simulink model "carSimACCLK"  (Simulink 10.2)
settings: Solver=ode23  StartTime=0.0  StopTime=80  FixedStep=1e-3  MaxStep=1e-2  RelTol=1e-3  EnableMultiTasking=on
libraries: simulink x5, dsparch4 x1
settings Model: LogicAnalyzerSignalOrdering=2c38dcc2-2ce4-44d7-bc47-ecfd3f78c9bc,43d34be1-2abe-4690-b550-79d99dd1860e,4a55a25e-455b-4f1c-be2e-1f375bbe41e4,4b197a40-1570-45d4-a952-fe9de0dc1ab5,12be2a9c-a868-4901-9855-7311f94e1c65,7a3363cb-5b35-4870-a861-6749fa4c6c84,d5c23654-3a48-4008-a3e4-0f09cca63f01,db4552fa-7eaf-453d-b285-63f4f7b0a5f4,005b0ed1-16df-4a19-95da-62a42ccf9ea3  Creator=hp  LastModifiedBy=11634
settings SolverCC: AlgebraicLoopSolver=LineSearch
settings DataIOCC: LimitDataPoints=on  SignalLoggingName=sigsOut
settings OptimizationCC: ExpressionDepthLimit=2147483647  InitFltsAndDblsToZero=on
settings DebuggingCC: SaveWithParameterizedLinksMsg=none  SignalResolutionControl=TryResolveAllWithWarning  MultiTaskDSMMsg=warning  MultiTaskCondExecSysMsg=none  StateNameClashWarn=warning
settings HardwareCC: TargetUnknown=on
settings GRTTargetCC: TargetFcnLib=ansi_tfl_tmw.mat

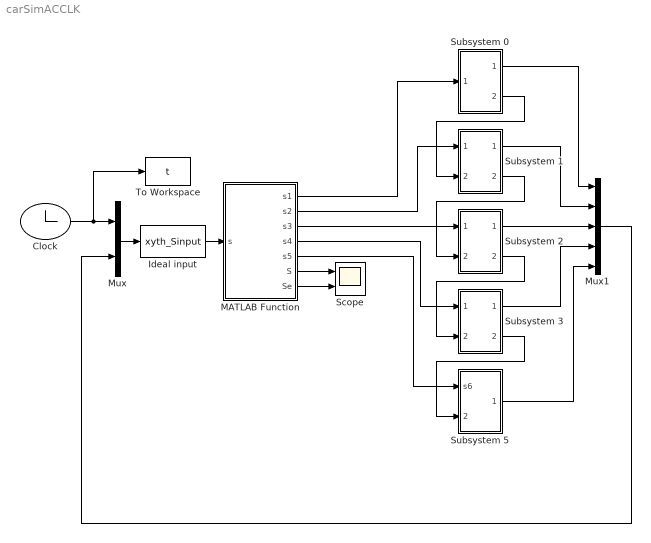
== system carSimACCLK ==
  Clock : Clock
  Ideal input : S-Function  FunctionName=xyth_Sinput  SFunctionDeploymentMode=off  EnableBusSupport=off
  MATLAB Function : MATLAB Function  TreatAsAtomicUnit=on
  Mux : Mux  Inputs=2
  Mux1 : Mux  Inputs=5
  Scope : Scope  NumInputPorts=2
  Subsystem 0 : Subsystem
  Subsystem 1 : Subsystem
  Subsystem 2 : Subsystem
  Subsystem 3 : Subsystem
  Subsystem 5 : Subsystem
  To Workspace : ToWorkspace  VariableName=t  SampleTime=-1
  wires:
  Clock/1 -> To Workspace/1, Mux/1
  Mux/1 -> Ideal input/1
  Ideal input/1 -> MATLAB Function/1(s)
  MATLAB Function/6(S) -> Scope/1
  MATLAB Function/7(Se) -> Scope/2
  MATLAB Function/2(s2) -> Subsystem 1/1(In1)
  Subsystem 1/1(Out1) -> Mux1/2
  MATLAB Function/1(s1) -> Subsystem 0/1(In1)
  Subsystem 0/1(Out1) -> Mux1/1
  Subsystem 0/2(Out2) -> Subsystem 1/2(In2)
  Subsystem 5/1(Out1) -> Mux1/5
  Mux1/1 -> Mux/2
  Subsystem 2/2(Out2) -> Subsystem 3/2(In2)
  Subsystem 2/1(Out1) -> Mux1/3
  Subsystem 3/1(Out1) -> Mux1/4
  MATLAB Function/4(s4) -> Subsystem 3/1(1)
  MATLAB Function/3(s3) -> Subsystem 2/1(In1)
  Subsystem 1/2(2) -> Subsystem 2/2(2)
  Subsystem 3/2(Out2) -> Subsystem 5/2(In2)
  MATLAB Function/5(s5) -> Subsystem 5/1(s6)

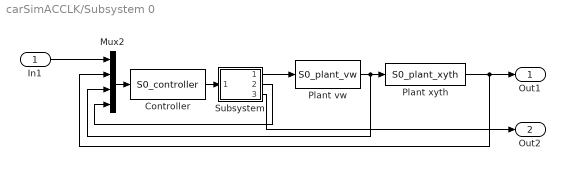
== system carSimACCLK/Subsystem 0 ==
  In1 : Inport
  Controller : S-Function  FunctionName=S0_controller  SFunctionDeploymentMode=off  EnableBusSupport=off
  Mux2 : Mux
  Plant vw : S-Function  FunctionName=S0_plant_vw  SFunctionDeploymentMode=off  EnableBusSupport=off
  Plant xyth : S-Function  FunctionName=S0_plant_xyth  SFunctionDeploymentMode=off  EnableBusSupport=off
  Subsystem : Subsystem
  Out1 : Outport
  Out2 : Outport  Port=2
  wires:
  Subsystem/1(Out1) -> Plant vw/1
  Subsystem/2(Out2) -> Mux2/4
  Subsystem/3(Out3) -> Out2/1
  Plant xyth/1 -> Mux2/2, Out1/1
  Mux2/1 -> Controller/1
  In1/1 -> Mux2/1
  Plant vw/1 -> Mux2/3, Plant xyth/1
  Controller/1 -> Subsystem/1(In1)

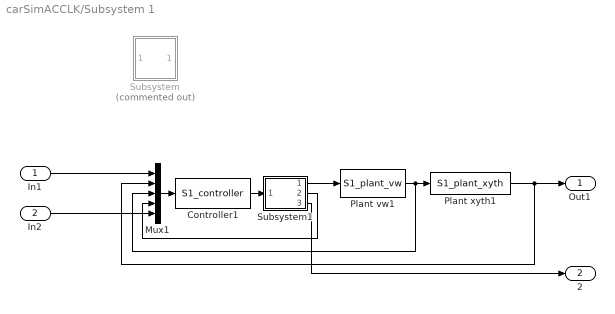
== system carSimACCLK/Subsystem 1 ==
  In1 : Inport
  In2 : Inport  Port=2
  Controller1 : S-Function  FunctionName=S1_controller  SFunctionDeploymentMode=off  EnableBusSupport=off
  Mux1 : Mux  Inputs=5
  Plant vw1 : S-Function  FunctionName=S1_plant_vw  SFunctionDeploymentMode=off  EnableBusSupport=off
  Plant xyth1 : S-Function  FunctionName=S1_plant_xyth  SFunctionDeploymentMode=off  EnableBusSupport=off
  Subsystem : Subsystem  Commented=on
  Subsystem1 : Subsystem
  Out1 : Outport
  2 : Outport  Port=2
  wires:
  Plant xyth1/1 -> Mux1/2, Out1/1
  In2/1 -> Mux1/5
  Plant vw1/1 -> Mux1/3, Plant xyth1/1
  Subsystem1/3(Out3) -> 2/1
  Subsystem1/1(Out1) -> Plant vw1/1
  Mux1/1 -> Controller1/1
  Controller1/1 -> Subsystem1/1(In1)
  Subsystem1/2(Out2) -> Mux1/4
  In1/1 -> Mux1/1

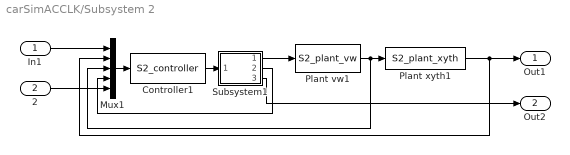
== system carSimACCLK/Subsystem 2 ==
  In1 : Inport
  2 : Inport  Port=2
  Controller1 : S-Function  FunctionName=S2_controller  SFunctionDeploymentMode=off  EnableBusSupport=off
  Mux1 : Mux  Inputs=5
  Plant vw1 : S-Function  FunctionName=S2_plant_vw  SFunctionDeploymentMode=off  EnableBusSupport=off
  Plant xyth1 : S-Function  FunctionName=S2_plant_xyth  SFunctionDeploymentMode=off  EnableBusSupport=off
  Subsystem1 : Subsystem
  Out1 : Outport
  Out2 : Outport  Port=2
  wires:
  Subsystem1/2(Out2) -> Mux1/4
  Controller1/1 -> Subsystem1/1(In1)
  Mux1/1 -> Controller1/1
  Subsystem1/1(Out1) -> Plant vw1/1
  Subsystem1/3(Out3) -> Out2/1
  Plant vw1/1 -> Mux1/3, Plant xyth1/1
  2/1 -> Mux1/5
  In1/1 -> Mux1/1
  Plant xyth1/1 -> Mux1/2, Out1/1

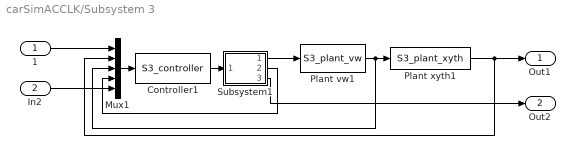
== system carSimACCLK/Subsystem 3 ==
  1 : Inport
  In2 : Inport  Port=2
  Controller1 : S-Function  FunctionName=S3_controller  SFunctionDeploymentMode=off  EnableBusSupport=off
  Mux1 : Mux  Inputs=5
  Plant vw1 : S-Function  FunctionName=S3_plant_vw  SFunctionDeploymentMode=off  EnableBusSupport=off
  Plant xyth1 : S-Function  FunctionName=S3_plant_xyth  SFunctionDeploymentMode=off  EnableBusSupport=off
  Subsystem1 : Subsystem
  Out1 : Outport
  Out2 : Outport  Port=2
  wires:
  Plant xyth1/1 -> Mux1/2, Out1/1
  1/1 -> Mux1/1
  In2/1 -> Mux1/5
  Plant vw1/1 -> Plant xyth1/1, Mux1/3
  Subsystem1/3(Out3) -> Out2/1
  Subsystem1/1(Out1) -> Plant vw1/1
  Mux1/1 -> Controller1/1
  Controller1/1 -> Subsystem1/1(In1)
  Subsystem1/2(Out2) -> Mux1/4

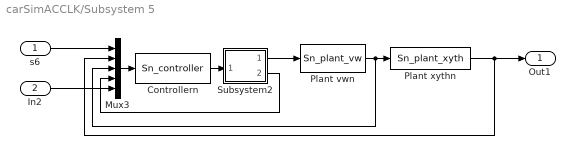
== system carSimACCLK/Subsystem 5 ==
  s6 : Inport
  In2 : Inport  Port=2
  Controllern : S-Function  FunctionName=Sn_controller  SFunctionDeploymentMode=off  EnableBusSupport=off
  Mux3 : Mux  Inputs=5
  Plant vwn : S-Function  FunctionName=Sn_plant_vw  SFunctionDeploymentMode=off  EnableBusSupport=off
  Plant xythn : S-Function  FunctionName=Sn_plant_xyth  SFunctionDeploymentMode=off  EnableBusSupport=off
  Subsystem2 : Subsystem
  Out1 : Outport
  wires:
  Subsystem2/1(Out1) -> Plant vwn/1
  Subsystem2/2(Out2) -> Mux3/4
  Mux3/1 -> Controllern/1
  Plant vwn/1 -> Mux3/3, Plant xythn/1
  Controllern/1 -> Subsystem2/1(In1)
  In2/1 -> Mux3/5
  Plant xythn/1 -> Mux3/2, Out1/1
  s6/1 -> Mux3/1

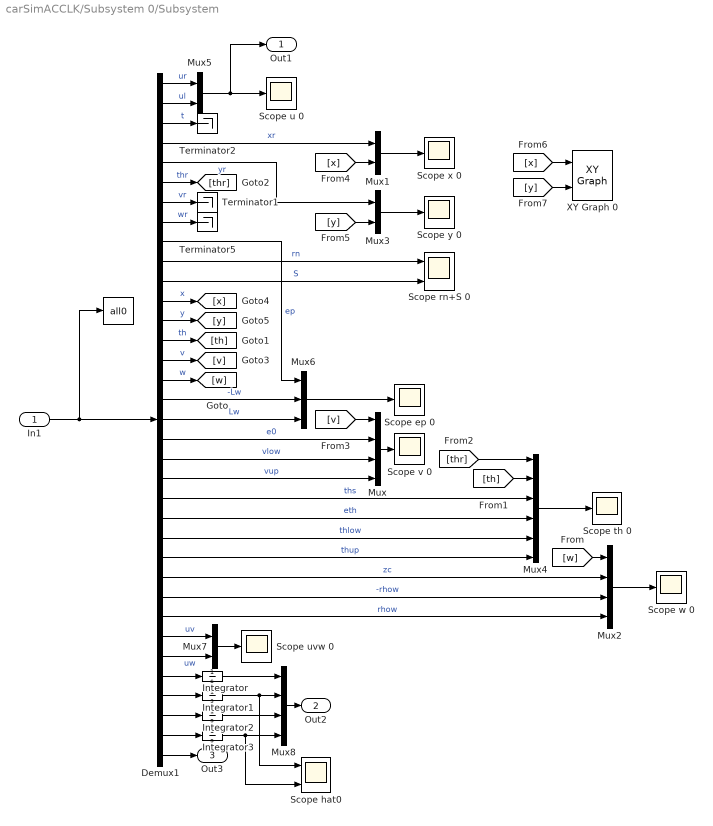
== system carSimACCLK/Subsystem 0/Subsystem ==
  In1 : Inport
  " " : ToWorkspace  VariableName=all0  SampleTime=-1
  Demux1 : Demux  Outputs=35
  Integrator : Integrator
  Integrator1 : Integrator  InitialCondition=0.1
  Integrator2 : Integrator
  Integrator3 : Integrator  InitialCondition=0.1
  Mux : Mux
  Mux{1,3,5,7} (4 alike) : Mux  Inputs=2
  Mux2 : Mux
  Mux4 : Mux  Inputs=6
  Mux6 : Mux  Inputs=3
  Mux8 : Mux
  Scope ep 0 : Scope
  Scope hat0 : Scope  NumInputPorts=2
  Scope rn+S 0 : Scope  NumInputPorts=2
  Scope th 0 : Scope
  Scope u 0 : Scope
  Scope uvw 0 : Scope
  Scope v 0 : Scope
  Scope w 0 : Scope
  Scope x 0 : Scope
  Scope y 0 : Scope
  Terminator1 : Terminator
  Terminator2 : Terminator
  Terminator5 : Terminator
  XY Graph 0 : simulink/Sinks/XY Graph  xmin=-400  xmax=400  ymin=-400  ymax=400  st=-1
  Out1 : Outport
  Out2 : Outport  Port=2
  Out3 : Outport  Port=3
  wires:
  In1/1 -> " "/1, Demux1/1
  Demux1/2 -> Mux5/2  "ul"
  Mux5/1 -> Scope u 0/1, Out1/1
  Demux1/1 -> Mux5/1  "ur"
  Mux3/1 -> Scope y 0/1
  Mux1/1 -> Scope x 0/1
  Demux1/6 -> [thr]  "thr"
  Demux1/8 -> Terminator5/1  "wr"
  Demux1/7 -> Terminator1/1  "vr"
  Demux1/3 -> Terminator2/1  "t"
  Demux1/4 -> Mux1/1  "xr"
  Demux1/5 -> Mux3/1  "yr"
  [x] -> Mux1/2
  [y] -> Mux3/2
  [x] -> XY Graph 0/1
  [y] -> XY Graph 0/2
  Demux1/10 -> Scope rn+S 0/1  "rn"
  Mux/1 -> Scope v 0/1
  Mux2/1 -> Scope w 0/1
  [w] -> Mux2/1
  [th] -> Mux4/2
  Mux6/1 -> Scope ep 0/1
  [thr] -> Mux4/1
  Demux1/13 -> [y]  "y"
  Demux1/28 -> Mux2/4  "rhow"
  Mux7/1 -> Scope uvw 0/1
  Demux1/29 -> Mux7/1  "uv"
  Demux1/12 -> [x]  "x"
  Demux1/15 -> [v]  "v"
  Demux1/14 -> [th]  "th"
  Demux1/17 -> Mux6/2  "-Lw"
  Demux1/27 -> Mux2/3  "-rhow"
  [v] -> Mux/1
  Demux1/26 -> Mux2/2  "zc"
  Demux1/22 -> Mux4/3  "ths"
  Demux1/23 -> Mux4/4  "eth"
  Demux1/19 -> Mux/2  "e0"
  Demux1/21 -> Mux/4  "vup"
  Demux1/16 -> [w]  "w"
  Demux1/25 -> Mux4/6  "thup"
  Demux1/24 -> Mux4/5  "thlow"
  Demux1/30 -> Mux7/2  "uw"
  Mux4/1 -> Scope th 0/1
  Demux1/20 -> Mux/3  "vlow"
  Demux1/9 -> Mux6/1  "ep"
  Demux1/18 -> Mux6/3  "Lw"
  Demux1/11 -> Scope rn+S 0/2  "S"
  Mux8/1 -> Out2/1
  Demux1/31 -> Integrator/1
  Demux1/32 -> Integrator1/1
  Integrator1/1 -> Mux8/2, Scope hat0/1
  Integrator/1 -> Mux8/1
  Integrator2/1 -> Mux8/3
  Demux1/33 -> Integrator2/1
  Integrator3/1 -> Mux8/4, Scope hat0/2
  Demux1/34 -> Integrator3/1
  Demux1/35 -> Out3/1

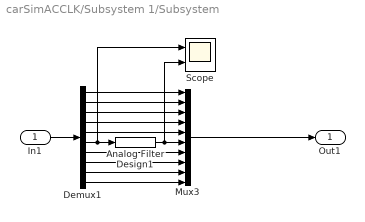
== system carSimACCLK/Subsystem 1/Subsystem ==
  In1 : Inport
  Analog Filter Design1 : dsparch4/Analog Filter Design  method=Butterworth  filttype=Lowpass  N=8  Wlo=50  Whi=80  Rp=2  Rs=40
  Demux1 : Demux  Outputs=10
  Mux3 : Mux  Inputs=10
  Scope : Scope  NumInputPorts=2
  Out1 : Outport
  wires:
  Demux1/1 -> Mux3/1
  Analog Filter Design1/1 -> Scope/2, Mux3/6
  Demux1/7 -> Mux3/7
  Mux3/1 -> Out1/1
  Demux1/4 -> Mux3/4
  Demux1/9 -> Mux3/9
  In1/1 -> Demux1/1
  Demux1/2 -> Mux3/2
  Demux1/3 -> Mux3/3
  Demux1/5 -> Mux3/5
  Demux1/10 -> Mux3/10
  Demux1/8 -> Mux3/8
  Demux1/6 -> Scope/1, Analog Filter Design1/1

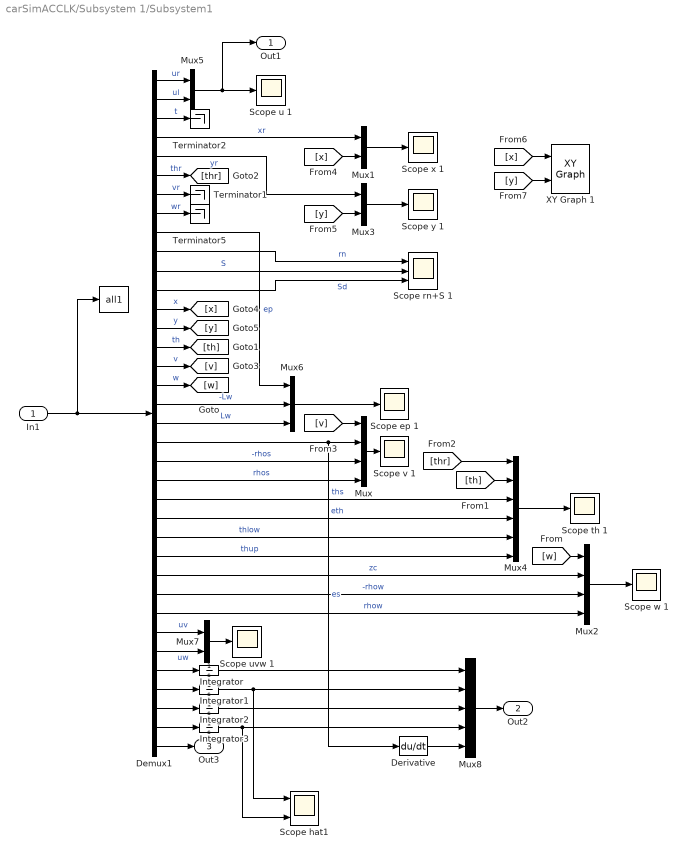
== system carSimACCLK/Subsystem 1/Subsystem1 ==
  In1 : Inport
  " " : ToWorkspace  VariableName=all1  SampleTime=-1
  Demux1 : Demux  Outputs=36
  Derivative : Derivative
  Integrator : Integrator
  Integrator1 : Integrator  InitialCondition=0.1
  Integrator2 : Integrator
  Integrator3 : Integrator  InitialCondition=0.1
  Mux : Mux
  Mux{1,3,5,7} (4 alike) : Mux  Inputs=2
  Mux2 : Mux
  Mux4 : Mux  Inputs=6
  Mux6 : Mux  Inputs=3
  Mux8 : Mux  Inputs=5
  Scope ep 1 : Scope
  Scope hat1 : Scope  NumInputPorts=2
  Scope rn+S 1 : Scope  NumInputPorts=3
  Scope th 1 : Scope
  Scope u 1 : Scope
  Scope uvw 1 : Scope
  Scope v 1 : Scope
  Scope w 1 : Scope
  Scope x 1 : Scope
  Scope y 1 : Scope
  Terminator1 : Terminator
  Terminator2 : Terminator
  Terminator5 : Terminator
  XY Graph 1 : simulink/Sinks/XY Graph  xmin=-400  xmax=400  ymin=-400  ymax=400  st=-1
  Out1 : Outport
  Out2 : Outport  Port=2
  Out3 : Outport  Port=3
  wires:
  Demux1/11 -> Scope rn+S 1/2  "S"
  Demux1/13 -> [x]  "x"
  Demux1/10 -> Scope rn+S 1/1  "rn"
  [y] -> XY Graph 1/2
  [x] -> XY Graph 1/1
  [y] -> Mux3/2
  [x] -> Mux1/2
  Demux1/5 -> Mux3/1  "yr"
  Demux1/4 -> Mux1/1  "xr"
  Demux1/3 -> Terminator2/1  "t"
  Demux1/7 -> Terminator1/1  "vr"
  Demux1/8 -> Terminator5/1  "wr"
  Demux1/6 -> [thr]  "thr"
  Mux1/1 -> Scope x 1/1
  Mux3/1 -> Scope y 1/1
  Demux1/1 -> Mux5/1  "ur"
  Mux5/1 -> Out1/1, Scope u 1/1
  Demux1/2 -> Mux5/2  "ul"
  In1/1 -> " "/1, Demux1/1
  Demux1/18 -> Mux6/2  "-Lw"
  Mux4/1 -> Scope th 1/1
  Mux/1 -> Scope v 1/1
  Demux1/30 -> Mux7/1  "uv"
  [w] -> Mux2/1
  [th] -> Mux4/2
  Demux1/16 -> [v]  "v"
  Mux6/1 -> Scope ep 1/1
  [thr] -> Mux4/1
  Demux1/21 -> Mux/3  "-rhos"
  Demux1/15 -> [th]  "th"
  [v] -> Mux/1
  Demux1/23 -> Mux4/3  "ths"
  Demux1/20 -> Mux/2, Derivative/1  "es"
  Demux1/25 -> Mux4/5  "thlow"
  Demux1/22 -> Mux/4  "rhos"
  Demux1/28 -> Mux2/3  "-rhow"
  Demux1/31 -> Mux7/2  "uw"
  Demux1/27 -> Mux2/2  "zc"
  Demux1/17 -> [w]  "w"
  Demux1/26 -> Mux4/6  "thup"
  Demux1/29 -> Mux2/4  "rhow"
  Demux1/19 -> Mux6/3  "Lw"
  Demux1/24 -> Mux4/4  "eth"
  Demux1/9 -> Mux6/1  "ep"
  Mux2/1 -> Scope w 1/1
  Mux7/1 -> Scope uvw 1/1
  Demux1/14 -> [y]  "y"
  Demux1/12 -> Scope rn+S 1/3  "Sd"
  Mux8/1 -> Out2/1
  Integrator/1 -> Mux8/1
  Demux1/32 -> Integrator/1
  Demux1/33 -> Integrator1/1
  Integrator1/1 -> Scope hat1/1, Mux8/2
  Demux1/36 -> Out3/1
  Demux1/34 -> Integrator2/1
  Demux1/35 -> Integrator3/1
  Integrator2/1 -> Mux8/3
  Integrator3/1 -> Scope hat1/2, Mux8/4
  Derivative/1 -> Mux8/5

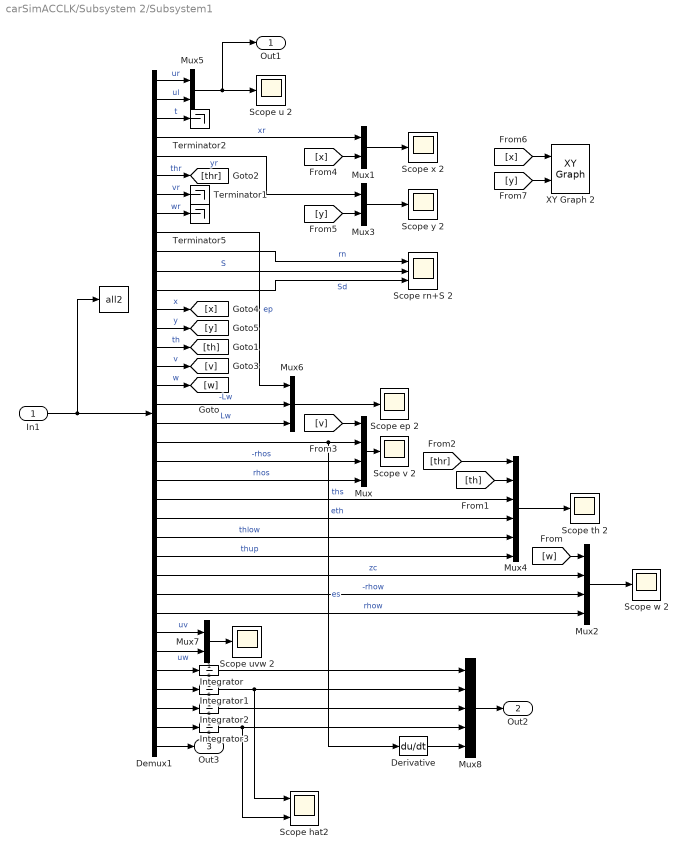
== system carSimACCLK/Subsystem 2/Subsystem1 ==
  In1 : Inport
  " " : ToWorkspace  VariableName=all2  SampleTime=-1
  Demux1 : Demux  Outputs=36
  Derivative : Derivative
  Integrator : Integrator
  Integrator1 : Integrator  InitialCondition=0.1
  Integrator2 : Integrator
  Integrator3 : Integrator  InitialCondition=0.1
  Mux : Mux
  Mux{1,3,5,7} (4 alike) : Mux  Inputs=2
  Mux2 : Mux
  Mux4 : Mux  Inputs=6
  Mux6 : Mux  Inputs=3
  Mux8 : Mux  Inputs=5
  Scope ep 2 : Scope
  Scope hat2 : Scope  NumInputPorts=2
  Scope rn+S 2 : Scope  NumInputPorts=3
  Scope th 2 : Scope
  Scope u 2 : Scope
  Scope uvw 2 : Scope
  Scope v 2 : Scope
  Scope w 2 : Scope
  Scope x 2 : Scope
  Scope y 2 : Scope
  Terminator1 : Terminator
  Terminator2 : Terminator
  Terminator5 : Terminator
  XY Graph 2 : simulink/Sinks/XY Graph  xmin=-400  xmax=400  ymin=-400  ymax=400  st=-1
  Out1 : Outport
  Out2 : Outport  Port=2
  Out3 : Outport  Port=3
  wires:
  Derivative/1 -> Mux8/5
  Integrator3/1 -> Mux8/4, Scope hat2/2
  Integrator2/1 -> Mux8/3
  Demux1/35 -> Integrator3/1
  Demux1/34 -> Integrator2/1
  Demux1/36 -> Out3/1
  Integrator1/1 -> Scope hat2/1, Mux8/2
  Demux1/33 -> Integrator1/1
  Demux1/32 -> Integrator/1
  Integrator/1 -> Mux8/1
  Mux8/1 -> Out2/1
  Demux1/12 -> Scope rn+S 2/3  "Sd"
  Demux1/14 -> [y]  "y"
  Mux7/1 -> Scope uvw 2/1
  Mux2/1 -> Scope w 2/1
  Demux1/9 -> Mux6/1  "ep"
  Demux1/24 -> Mux4/4  "eth"
  Demux1/19 -> Mux6/3  "Lw"
  Demux1/29 -> Mux2/4  "rhow"
  Demux1/26 -> Mux4/6  "thup"
  Demux1/17 -> [w]  "w"
  Demux1/27 -> Mux2/2  "zc"
  Demux1/31 -> Mux7/2  "uw"
  Demux1/28 -> Mux2/3  "-rhow"
  Demux1/22 -> Mux/4  "rhos"
  Demux1/25 -> Mux4/5  "thlow"
  Demux1/20 -> Derivative/1, Mux/2  "es"
  Demux1/23 -> Mux4/3  "ths"
  [v] -> Mux/1
  Demux1/15 -> [th]  "th"
  Demux1/21 -> Mux/3  "-rhos"
  [thr] -> Mux4/1
  Mux6/1 -> Scope ep 2/1
  Demux1/16 -> [v]  "v"
  [th] -> Mux4/2
  [w] -> Mux2/1
  Demux1/30 -> Mux7/1  "uv"
  Mux/1 -> Scope v 2/1
  Mux4/1 -> Scope th 2/1
  Demux1/18 -> Mux6/2  "-Lw"
  In1/1 -> Demux1/1, " "/1
  Demux1/2 -> Mux5/2  "ul"
  Mux5/1 -> Scope u 2/1, Out1/1
  Demux1/1 -> Mux5/1  "ur"
  Mux3/1 -> Scope y 2/1
  Mux1/1 -> Scope x 2/1
  Demux1/6 -> [thr]  "thr"
  Demux1/8 -> Terminator5/1  "wr"
  Demux1/7 -> Terminator1/1  "vr"
  Demux1/3 -> Terminator2/1  "t"
  Demux1/4 -> Mux1/1  "xr"
  Demux1/5 -> Mux3/1  "yr"
  [x] -> Mux1/2
  [y] -> Mux3/2
  [x] -> XY Graph 2/1
  [y] -> XY Graph 2/2
  Demux1/10 -> Scope rn+S 2/1  "rn"
  Demux1/13 -> [x]  "x"
  Demux1/11 -> Scope rn+S 2/2  "S"

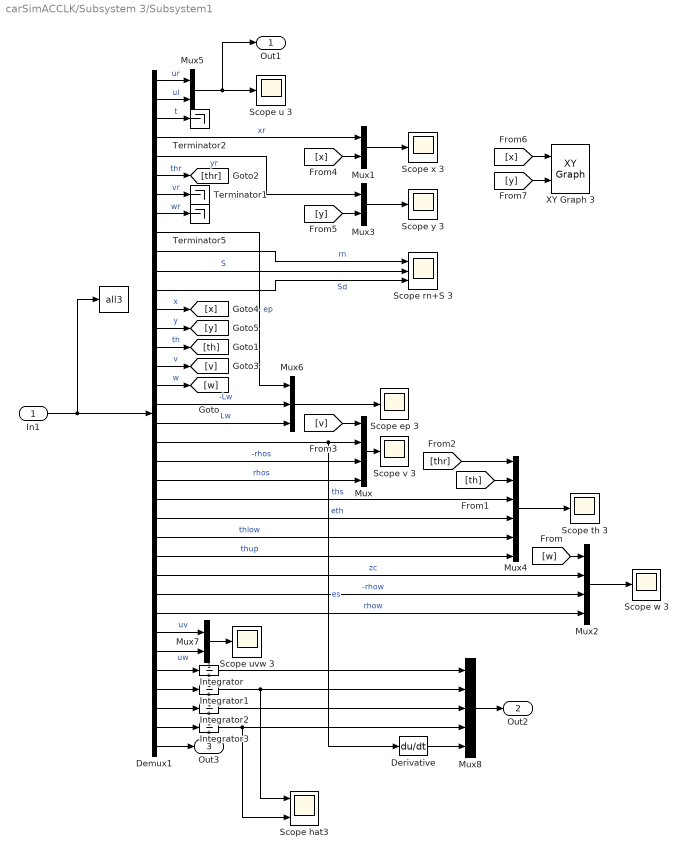
== system carSimACCLK/Subsystem 3/Subsystem1 ==
  In1 : Inport
  " " : ToWorkspace  VariableName=all3  SampleTime=-1
  Demux1 : Demux  Outputs=36
  Derivative : Derivative
  Integrator : Integrator
  Integrator1 : Integrator  InitialCondition=0.1
  Integrator2 : Integrator
  Integrator3 : Integrator  InitialCondition=0.1
  Mux : Mux
  Mux{1,3,5,7} (4 alike) : Mux  Inputs=2
  Mux2 : Mux
  Mux4 : Mux  Inputs=6
  Mux6 : Mux  Inputs=3
  Mux8 : Mux  Inputs=5
  Scope ep 3 : Scope
  Scope hat3 : Scope  NumInputPorts=2
  Scope rn+S 3 : Scope  NumInputPorts=3
  Scope th 3 : Scope
  Scope u 3 : Scope
  Scope uvw 3 : Scope
  Scope v 3 : Scope
  Scope w 3 : Scope
  Scope x 3 : Scope
  Scope y 3 : Scope
  Terminator1 : Terminator
  Terminator2 : Terminator
  Terminator5 : Terminator
  XY Graph 3 : simulink/Sinks/XY Graph  xmin=-400  xmax=400  ymin=-400  ymax=400  st=-1
  Out1 : Outport
  Out2 : Outport  Port=2
  Out3 : Outport  Port=3
  wires:
  Demux1/11 -> Scope rn+S 3/2  "S"
  Demux1/13 -> [x]  "x"
  Demux1/10 -> Scope rn+S 3/1  "rn"
  [y] -> XY Graph 3/2
  [x] -> XY Graph 3/1
  [y] -> Mux3/2
  [x] -> Mux1/2
  Demux1/5 -> Mux3/1  "yr"
  Demux1/4 -> Mux1/1  "xr"
  Demux1/3 -> Terminator2/1  "t"
  Demux1/7 -> Terminator1/1  "vr"
  Demux1/8 -> Terminator5/1  "wr"
  Demux1/6 -> [thr]  "thr"
  Mux1/1 -> Scope x 3/1
  Mux3/1 -> Scope y 3/1
  Demux1/1 -> Mux5/1  "ur"
  Mux5/1 -> Out1/1, Scope u 3/1
  Demux1/2 -> Mux5/2  "ul"
  In1/1 -> " "/1, Demux1/1
  Demux1/18 -> Mux6/2  "-Lw"
  Mux4/1 -> Scope th 3/1
  Mux/1 -> Scope v 3/1
  Demux1/30 -> Mux7/1  "uv"
  [w] -> Mux2/1
  [th] -> Mux4/2
  Demux1/16 -> [v]  "v"
  Mux6/1 -> Scope ep 3/1
  [thr] -> Mux4/1
  Demux1/21 -> Mux/3  "-rhos"
  Demux1/15 -> [th]  "th"
  [v] -> Mux/1
  Demux1/23 -> Mux4/3  "ths"
  Demux1/20 -> Mux/2, Derivative/1  "es"
  Demux1/25 -> Mux4/5  "thlow"
  Demux1/22 -> Mux/4  "rhos"
  Demux1/28 -> Mux2/3  "-rhow"
  Demux1/31 -> Mux7/2  "uw"
  Demux1/27 -> Mux2/2  "zc"
  Demux1/17 -> [w]  "w"
  Demux1/26 -> Mux4/6  "thup"
  Demux1/29 -> Mux2/4  "rhow"
  Demux1/19 -> Mux6/3  "Lw"
  Demux1/24 -> Mux4/4  "eth"
  Demux1/9 -> Mux6/1  "ep"
  Mux2/1 -> Scope w 3/1
  Mux7/1 -> Scope uvw 3/1
  Demux1/14 -> [y]  "y"
  Demux1/12 -> Scope rn+S 3/3  "Sd"
  Mux8/1 -> Out2/1
  Integrator/1 -> Mux8/1
  Demux1/32 -> Integrator/1
  Demux1/33 -> Integrator1/1
  Integrator1/1 -> Scope hat3/1, Mux8/2
  Demux1/36 -> Out3/1
  Demux1/34 -> Integrator2/1
  Demux1/35 -> Integrator3/1
  Integrator2/1 -> Mux8/3
  Integrator3/1 -> Scope hat3/2, Mux8/4
  Derivative/1 -> Mux8/5

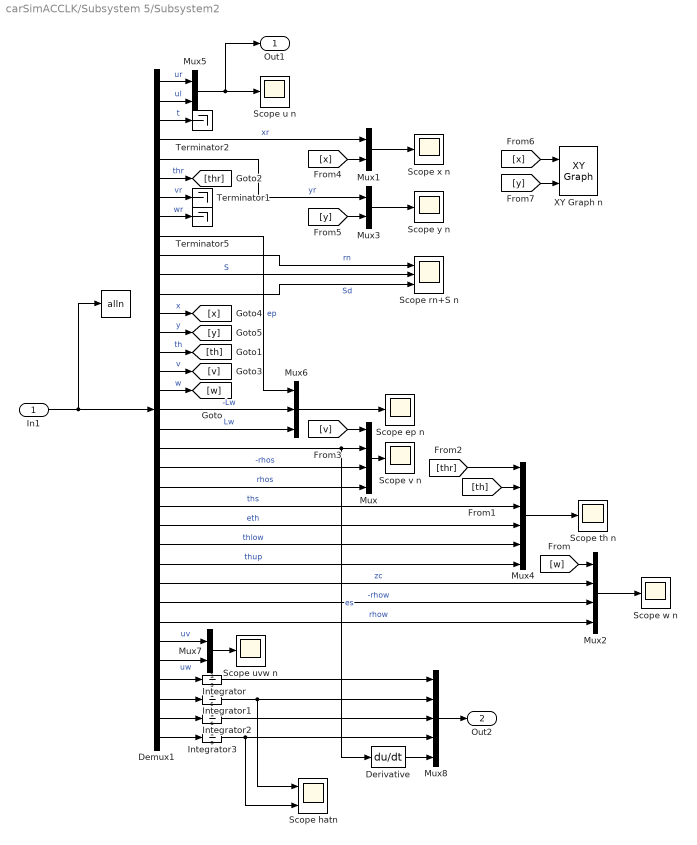
== system carSimACCLK/Subsystem 5/Subsystem2 ==
  In1 : Inport
  " " : ToWorkspace  VariableName=alln  SampleTime=-1
  Demux1 : Demux  Outputs=35
  Derivative : Derivative
  Integrator : Integrator
  Integrator1 : Integrator  InitialCondition=0.1
  Integrator2 : Integrator
  Integrator3 : Integrator  InitialCondition=0.1
  Mux : Mux
  Mux{1,3,5,7} (4 alike) : Mux  Inputs=2
  Mux2 : Mux
  Mux4 : Mux  Inputs=6
  Mux6 : Mux  Inputs=3
  Mux8 : Mux  Inputs=5
  Scope ep n : Scope
  Scope hatn : Scope  NumInputPorts=2
  Scope rn+S n : Scope  NumInputPorts=3
  Scope th n : Scope
  Scope u n : Scope
  Scope uvw n : Scope
  Scope v n : Scope
  Scope w n : Scope
  Scope x n : Scope
  Scope y n : Scope
  Terminator1 : Terminator
  Terminator2 : Terminator
  Terminator5 : Terminator
  XY Graph n : simulink/Sinks/XY Graph  xmin=-400  xmax=400  ymin=-400  ymax=400  st=-1
  Out1 : Outport
  Out2 : Outport  Port=2
  wires:
  In1/1 -> " "/1, Demux1/1
  Demux1/2 -> Mux5/2  "ul"
  Mux5/1 -> Scope u n/1, Out1/1
  Demux1/1 -> Mux5/1  "ur"
  Mux3/1 -> Scope y n/1
  Mux1/1 -> Scope x n/1
  Demux1/6 -> [thr]  "thr"
  Demux1/8 -> Terminator5/1  "wr"
  Demux1/7 -> Terminator1/1  "vr"
  Demux1/3 -> Terminator2/1  "t"
  Demux1/4 -> Mux1/1  "xr"
  Demux1/5 -> Mux3/1  "yr"
  [x] -> Mux1/2
  [y] -> Mux3/2
  [x] -> XY Graph n/1
  [y] -> XY Graph n/2
  Demux1/10 -> Scope rn+S n/1  "rn"
  Demux1/11 -> Scope rn+S n/2  "S"
  Mux7/1 -> Scope uvw n/1
  Demux1/14 -> [y]  "y"
  Demux1/25 -> Mux4/5  "thlow"
  Mux/1 -> Scope v n/1
  Demux1/9 -> Mux6/1  "ep"
  [th] -> Mux4/2
  Demux1/21 -> Mux/3  "-rhos"
  Mux4/1 -> Scope th n/1
  Demux1/26 -> Mux4/6  "thup"
  Demux1/22 -> Mux/4  "rhos"
  Demux1/27 -> Mux2/2  "zc"
  Demux1/17 -> [w]  "w"
  Demux1/24 -> Mux4/4  "eth"
  [v] -> Mux/1
  [thr] -> Mux4/1
  Demux1/23 -> Mux4/3  "ths"
  Demux1/30 -> Mux7/1  "uv"
  Demux1/19 -> Mux6/3  "Lw"
  Mux2/1 -> Scope w n/1
  Demux1/31 -> Mux7/2  "uw"
  Demux1/16 -> [v]  "v"
  [w] -> Mux2/1
  Demux1/15 -> [th]  "th"
  Demux1/13 -> [x]  "x"
  Demux1/20 -> Derivative/1, Mux/2  "es"
  Demux1/29 -> Mux2/4  "rhow"
  Integrator1/1 -> Scope hatn/1, Mux8/2
  Integrator/1 -> Mux8/1
  Demux1/18 -> Mux6/2  "-Lw"
  Demux1/32 -> Integrator/1
  Mux6/1 -> Scope ep n/1
  Demux1/33 -> Integrator1/1
  Mux8/1 -> Out2/1
  Demux1/28 -> Mux2/3  "-rhow"
  Demux1/12 -> Scope rn+S n/3  "Sd"
  Demux1/34 -> Integrator2/1
  Demux1/35 -> Integrator3/1
  Integrator2/1 -> Mux8/3
  Integrator3/1 -> Scope hatn/2, Mux8/4
  Derivative/1 -> Mux8/5

== matlab function MATLAB Function ==
  data: s input double; s1 output double; s2 output double; s3 output double; s4 output double; s5 output double; S output double; Se output double
function [s1,s2,s3,s4,s5,S,Se] = fcn(s)

t = s(1);
ni = 1; s1 = [t;s(ni*9-7:ni*9+1)];%2~10
ni = 2; s2 = [t;s(ni*9-7:ni*9+1)];%11~19
ni = 3; s3 = [t;s(ni*9-7:ni*9+1)];%20~28
ni = 4; s4 = [t;s(ni*9-7:ni*9+1)];%29~37
ni = 5; s5 = [t;s(ni*9-7:ni*9+1)];%38~46
S = [s(9),s(18),s(27),s(36),s(45)];
Se = [s(19),s(28),s(37),s(46)];
